simulink model "wykresy"  (R2018a)
settings: Solver=ode45  StartTime=0.0  StopTime=10.0  MaxStep=0.05  RelTol=1e-3  AbsTol=1e-6  EnableMultiTasking=on
values from neighbouring files (symbols this model uses):
  A1 = 1    [Lab06.m]
  a1 = (Aw1.*sqrt(2.*g.*h1max))/(h1max)    [Lab06.m]
  A2 = 2    [Lab06.m]
  a2 = (Aw2.*sqrt(2.*g.*h2max))/(h2max)    [Lab06.m]
  dfwe1 = 0    [Lab06.m]
  dfwe2 = 0.1*fwe2max    [Lab06.m]
  fwe1 = 0.2.*fwe1max    [Lab06.m]
  fwe2 = fwe2tab(i)    [Lab06.m]
  h01 = fwe1./a1    [Lab06.m]
  h02 = (fwe2+fwe1)./a2    [Lab06.m]
  t0 = 2    [Lab06.m]
settings Model: Creator=LAB320-1552  LastModifiedBy=johnb
settings SolverCC: AutoScaleAbsTol=off
settings DataIOCC: LimitDataPoints=on  SaveFormat=Array
settings OptimizationCC: LifeSpan=inf
settings DebuggingCC: UnderspecifiedInitializationDetection=Classic  MergeDetectMultiDrivingBlocksExec=none  StateNameClashWarn=warning  SFUnexpectedBacktrackingDiag=warning  SFNoUnconditionalDefaultTransitionDiag=warning  SFExecutionAtInitializationDiag=none
settings HardwareCC: ProdBitPerPointer=32  ProdBitPerSizeT=32  ProdBitPerPtrDiffT=32  ProdLargestAtomicFloat=None  ProdIntDivRoundTo=Undefined  ProdEndianess=Unspecified  ProdWordSize=32  ProdHWDeviceType=32-bit Generic
settings ModelReferenceCC: PropagateSignalLabelsOutOfModel=off
settings CodeAppCC: StateflowObjectComments=on
settings GRTTargetCC: TargetLangStandard=C89/C90 (ANSI)  GeneratePreprocessorConditionals=Disable all
settings ConfigComp: CovMetricSettings=dw  CovHtmlReporting=on  CovSaveCumulativeToWorkspaceVar=on  CovSaveSingleToWorkspaceVar=on  CovExternalEMLEnable=off

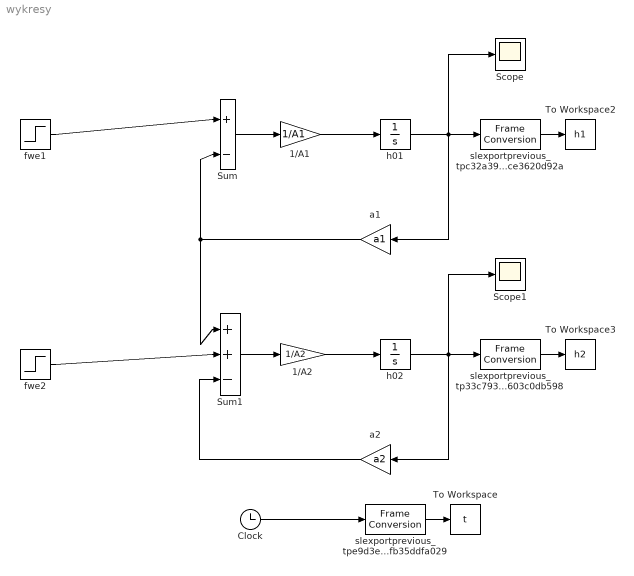
== system wykresy ==
  1/A1 : Gain  Gain=1/A1
  1/A2 : Gain  Gain=1/A2
  Clock : Clock
  Scope : Scope
  Scope1 : Scope
  Sum : Sum  Inputs=|+-
  Sum1 : Sum  Inputs=|++-
  To Workspace : ToWorkspace  VariableName=t  SampleTime=-1
  To Workspace2 : ToWorkspace  VariableName=h1  SampleTime=-1
  To Workspace3 : ToWorkspace  VariableName=h2  SampleTime=-1
  a1 : Gain  Gain=a1
  a2 : Gain  Gain=a2
  fwe1 : Step  Time=t0  Before=fwe1  After=fwe1+dfwe1  SampleTime=0
  fwe2 : Step  Time=t0  Before=fwe2  After=fwe2+dfwe2  SampleTime=0
  h01 : Integrator  InitialCondition=h01
  h02 : Integrator  InitialCondition=h02
  slexportprevious_tp33c7932a_40ae_4cc8_8a03_88603c0db598 : FrameConversion  OutFrame=Sample-based
  slexportprevious_tpc32a395d_d11c_4d8e_83cd_08ce3620d92a : FrameConversion  OutFrame=Sample-based
  slexportprevious_tpe9d3e0ca_1076_406b_bbce_efb35ddfa029 : FrameConversion  OutFrame=Sample-based
  wires:
  fwe1/1 -> Sum/1
  Sum/1 -> 1/A1/1
  1/A1/1 -> h01/1
  h01/1 -> Scope/1, a1/1, slexportprevious_tpc32a395d_d11c_4d8e_83cd_08ce3620d92a/1
  a1/1 -> Sum/2, Sum1/1
  Sum1/1 -> 1/A2/1
  1/A2/1 -> h02/1
  h02/1 -> Scope1/1, a2/1, slexportprevious_tp33c7932a_40ae_4cc8_8a03_88603c0db598/1
  fwe2/1 -> Sum1/2
  a2/1 -> Sum1/3
  Clock/1 -> slexportprevious_tpe9d3e0ca_1076_406b_bbce_efb35ddfa029/1
  slexportprevious_tpe9d3e0ca_1076_406b_bbce_efb35ddfa029/1 -> To Workspace/1
  slexportprevious_tpc32a395d_d11c_4d8e_83cd_08ce3620d92a/1 -> To Workspace2/1
  slexportprevious_tp33c7932a_40ae_4cc8_8a03_88603c0db598/1 -> To Workspace3/1
